simulink model "sampleModel1479_sub_sub"  (R2023a)
settings: Solver=VariableStepAuto  StartTime=0.0  StopTime=10.0  RelTol=1e-3
libraries: hdlsllib x6
settings Model: Creator=user1  LastModifiedBy=user1
settings OptimizationCC: BlockReduction=off  ConditionallyExecuteInputs=off

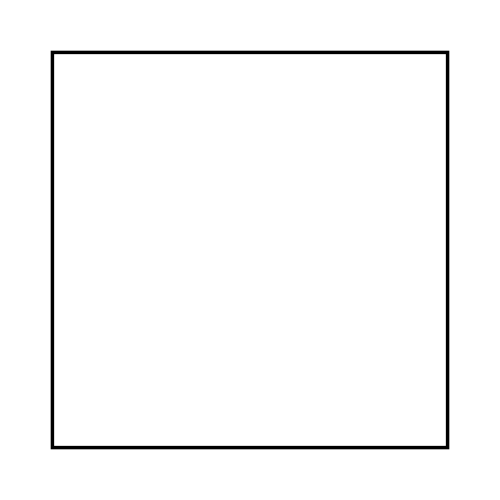
[thumbnail: Simulink's stored preview of the top-level diagram]
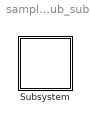
== system sampleModel1479_sub_sub ==
  Subsystem : Subsystem

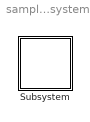
== system sampleModel1479_sub_sub/Subsystem ==
  Subsystem : Subsystem

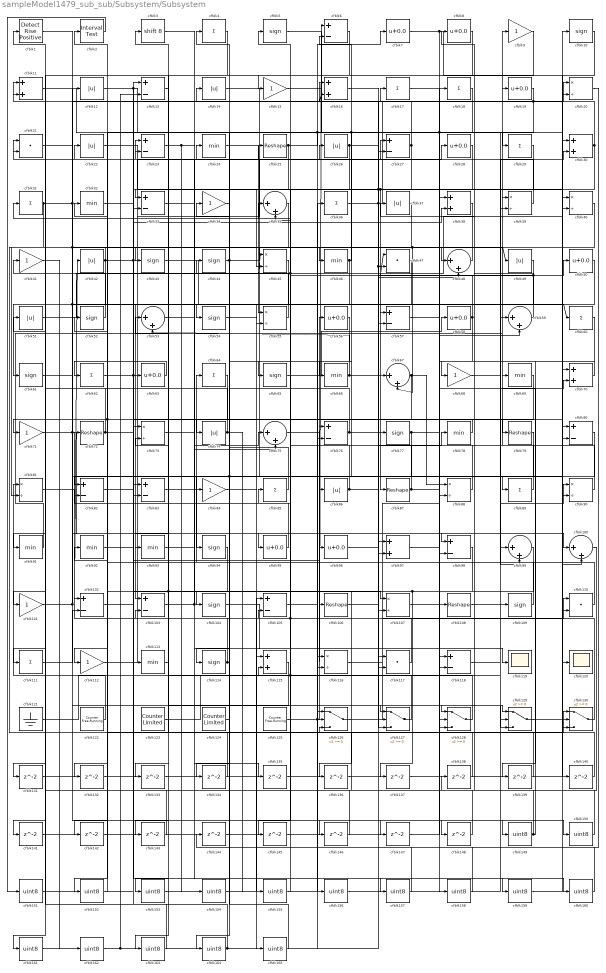
== system sampleModel1479_sub_sub/Subsystem/Subsystem ==
  cfblk1 : hdlsllib/Logic and Bit Operations/Detect Rise Positive  vinit=0  OutDataTypeStr=uint8
  cfblk{5,10,43..44,52,54,61,65,77,94,104,109,114} (13 alike) : Signum
  cfblk{35,48,53,59,67,75,99..100} (8 alike) : Sum  Inputs=|++  OutDataTypeStr=uint8
  cfblk{9,15,34,41,68,71,84,101,112} (9 alike) : Gain  OutDataTypeStr=uint8
  cfblk{6,13,23,27,33,57,76,80,82..83,98,102..103,105,118} (15 alike) : Sum  Inputs=+-  OutDataTypeStr=uint8
  cfblk{25,72,79,87,106,108} (6 alike) : Reshape
  cfblk{20,39..40,45,55,73,81,88,90,107,116} (11 alike) : Product  Inputs=*/  OutDataTypeStr=uint8  RndMeth=Zero  SaturateOnIntegerOverflow=on
  cfblk{11,16,30,38,70,97,115} (7 alike) : Sum  OutDataTypeStr=uint8
  cfblk{21,47,110,117} (4 alike) : DotProduct  OutDataTypeStr=uint8
  cfblk{4,17..18,29,31,36,60,62,64,85,89,111} (12 alike) : Sum  Inputs=+  OutDataTypeStr=uint8
  cfblk{24,32,46,66,69,78,91..93,113} (10 alike) : MinMax  OutDataTypeStr=uint8
  cfblk119 : Scope
  cfblk{12,14,22,26,37,42,49,51,74,86} (10 alike) : Abs  OutDataTypeStr=uint8  SaturateOnIntegerOverflow=off
  cfblk120 : Scope
  cfblk121 : Ground
  cfblk122 : hdlsllib/Sources/Counter Free-Running  NumBits=16  tsamp=-1
  cfblk123 : hdlsllib/Sources/Counter Limited  uplimit=7  tsamp=-1
  cfblk124 : hdlsllib/Sources/Counter Limited  uplimit=7  tsamp=-1
  cfblk125 : hdlsllib/Sources/Counter Free-Running  NumBits=16  tsamp=-1
  cfblk{126..130} (5 alike) : Switch  OutDataTypeStr=uint8  SaturateOnIntegerOverflow=off  InputSameDT=off
  cfblk{131..148} (18 alike) : Delay  SampleTime=1
  cfblk{149..165} (17 alike) : DataTypeConversion  OutDataTypeStr=uint8  SaturateOnIntegerOverflow=off  RndMeth=Floor
  cfblk{7..8,19,28,50,56,58,63,95..96} (10 alike) : Bias  Bias=0.0  SaturateOnIntegerOverflow=off
  cfblk2 : hdlsllib/Logic and Bit Operations/Interval Test  IntervalClosedRight=on  uplimit=0.5  IntervalClosedLeft=on  lowlimit=-0.5  OutDataTypeStr=uint8
  cfblk3 : ArithShift  BitShiftNumber=8
  wires:
  cfblk165/1 -> cfblk34/1
  cfblk54/1 -> cfblk165/1
  cfblk164/1 -> cfblk27/2, cfblk13/1
  cfblk163/1 -> cfblk41/1
  cfblk162/1 -> cfblk116/2, cfblk13/2
  cfblk161/1 -> cfblk97/2
  cfblk160/1 -> cfblk97/1
  cfblk73/1 -> cfblk160/1
  cfblk159/1 -> cfblk40/2
  cfblk97/1 -> cfblk159/1
  cfblk158/1 -> cfblk105/2
  cfblk104/1 -> cfblk158/1
  cfblk157/1 -> cfblk105/1
  cfblk32/1 -> cfblk157/1
  cfblk156/1 -> cfblk109/1
  cfblk105/1 -> cfblk156/1
  cfblk155/1 -> cfblk115/2
  cfblk154/1 -> cfblk115/1
  cfblk153/1 -> cfblk116/1
  cfblk115/1 -> cfblk153/1
  cfblk152/1 -> cfblk2/1
  cfblk37/1 -> cfblk152/1
  cfblk151/1 -> cfblk63/1
  cfblk2/1 -> cfblk151/1
  cfblk150/1 -> cfblk1/1
  cfblk147/1 -> cfblk150/1
  cfblk149/1 -> cfblk8/1, cfblk69/1
  cfblk148/1 -> cfblk126/3
  cfblk84/1 -> cfblk147/1
  cfblk146/1 -> cfblk73/1
  cfblk92/1 -> cfblk146/1
  cfblk145/1 -> cfblk88/2
  cfblk144/1 -> cfblk38/1
  cfblk20/1 -> cfblk144/1
  cfblk143/1 -> cfblk83/1
  cfblk13/1 -> cfblk143/1
  cfblk142/1 -> cfblk98/2
  cfblk141/1 -> cfblk67/1
  cfblk6/1 -> cfblk141/1
  cfblk140/1 -> cfblk126/1
  cfblk129/1 -> cfblk140/1
  cfblk139/1 -> cfblk103/2
  cfblk60/1 -> cfblk139/1
  cfblk138/1 -> cfblk35/2
  cfblk100/1 -> cfblk138/1
  cfblk137/1 -> cfblk110/2
  cfblk136/1 -> cfblk30/1
  cfblk135/1 -> cfblk70/1
  cfblk53/1 -> cfblk135/1
  cfblk134/1 -> cfblk82/2
  cfblk133/1 -> cfblk39/2
  cfblk132/1 -> cfblk40/1
  cfblk18/1 -> cfblk132/1
  cfblk131/1 -> cfblk57/2
  cfblk52/1 -> cfblk21/2
  cfblk118/1 -> cfblk99/1
  cfblk103/1 -> cfblk27/1, cfblk127/3
  cfblk19/1 -> cfblk76/2, cfblk54/1, cfblk86/1, cfblk16/2
  cfblk80/1 -> cfblk133/1, cfblk134/1
  cfblk124/1 -> cfblk44/1
  cfblk67/1 -> cfblk88/1, cfblk131/1
  cfblk4/1 -> cfblk43/1
  cfblk15/1 -> cfblk118/1, cfblk99/2
  cfblk58/1 -> cfblk25/1, cfblk128/2
  cfblk31/1 -> cfblk84/1, cfblk49/1, cfblk16/1, cfblk81/2
  cfblk111/1 -> cfblk102/2
  cfblk75/1 -> cfblk76/1
  cfblk10/1 -> cfblk130/3
  cfblk69/1 -> cfblk112/1, cfblk161/1
  cfblk46/1 -> cfblk6/2, cfblk83/2
  cfblk28/1 -> cfblk47/2, cfblk117/2, cfblk126/2
  cfblk79/1 -> cfblk82/1
  cfblk114/1 -> cfblk14/1, cfblk92/1
  cfblk41/1 -> cfblk162/1
  cfblk35/1 -> cfblk111/1
  cfblk126/1 -> cfblk110/1
  cfblk68/1 -> cfblk30/2
  cfblk107/1 -> cfblk129/1
  cfblk36/1 -> cfblk19/1, cfblk118/2
  cfblk48/1 -> cfblk46/1
  cfblk106/1 -> cfblk20/1
  cfblk3/1 -> cfblk107/1
  cfblk78/1 -> cfblk71/1
  cfblk7/1 -> cfblk100/2, cfblk129/3
  cfblk23/1 -> cfblk75/2, cfblk154/1
  cfblk5/1 -> cfblk120/1
  cfblk61/1 -> cfblk100/1
  cfblk17/1 -> cfblk108/1
  cfblk70/1 -> cfblk68/1
  cfblk43/1 -> cfblk55/2
  cfblk98/1 -> cfblk114/1
  cfblk40/1 -> cfblk67/2, cfblk66/1
  cfblk21/1 -> cfblk60/1, cfblk128/3
  cfblk101/1 -> cfblk12/1, cfblk148/1
  cfblk57/1 -> cfblk79/1
  cfblk108/1 -> cfblk90/1
  cfblk22/1 -> cfblk80/1, cfblk117/1
  cfblk66/1 -> cfblk53/2, cfblk128/1
  cfblk94/1 -> cfblk142/1, cfblk163/1
  cfblk109/1 -> cfblk52/1
  cfblk25/1 -> cfblk7/1, cfblk45/2
  cfblk45/1 -> cfblk74/1
  cfblk113/1 -> cfblk73/2
  cfblk16/1 -> cfblk98/1
  cfblk130/1 -> cfblk53/1
  cfblk81/1 -> cfblk102/1
  cfblk99/1 -> cfblk136/1, cfblk137/1
  cfblk59/1 -> cfblk47/1, cfblk37/1
  cfblk82/1 -> cfblk113/1
  cfblk27/1 -> cfblk11/2, cfblk127/2
  cfblk34/1 -> cfblk164/1
  cfblk85/1 -> cfblk4/1
  cfblk49/1 -> cfblk65/1
  cfblk11/1 -> cfblk130/2
  cfblk9/1 -> cfblk15/1
  cfblk96/1 -> cfblk50/1
  cfblk1/1 -> cfblk149/1
  cfblk93/1 -> cfblk75/1
  cfblk88/1 -> cfblk31/1
  cfblk74/1 -> cfblk51/1, cfblk155/1
  cfblk77/1 -> cfblk70/2, cfblk107/2
  cfblk86/1 -> cfblk78/1, cfblk23/2
  cfblk102/1 -> cfblk96/1
  cfblk72/1 -> cfblk11/1, cfblk90/2
  cfblk63/1 -> cfblk62/1
  cfblk76/1 -> cfblk77/1, cfblk24/1
  cfblk29/1 -> cfblk57/1, cfblk33/2
  cfblk87/1 -> cfblk35/1, cfblk59/2
  cfblk62/1 -> cfblk26/1, cfblk20/2
  cfblk24/1 -> cfblk55/1
  cfblk30/1 -> cfblk17/1, cfblk145/1
  cfblk26/1 -> cfblk33/1, cfblk48/2
  cfblk123/1 -> cfblk59/1
  cfblk95/1 -> cfblk72/1
  cfblk51/1 -> cfblk10/1
  cfblk65/1 -> cfblk58/1
  cfblk64/1 -> cfblk101/1
  cfblk33/1 -> cfblk119/1
  cfblk55/1 -> cfblk32/1
  cfblk89/1 -> cfblk23/1
  cfblk116/1 -> cfblk18/1
  cfblk8/1 -> cfblk93/1
  cfblk50/1 -> cfblk61/1
  cfblk12/1 -> cfblk29/1, cfblk80/2
  cfblk121/1 -> cfblk36/1
  cfblk83/1 -> cfblk94/1
  cfblk39/1 -> cfblk22/1
  cfblk128/1 -> cfblk5/1, cfblk45/1, cfblk3/1
  cfblk127/1 -> cfblk56/1
  cfblk47/1 -> cfblk103/1
  cfblk38/1 -> cfblk87/1
  cfblk90/1 -> cfblk39/1
  cfblk14/1 -> cfblk89/1
  cfblk112/1 -> cfblk28/1
  cfblk42/1 -> cfblk38/2, cfblk106/1, cfblk130/1, cfblk91/1
  cfblk125/1 -> cfblk6/1, cfblk127/1
  cfblk56/1 -> cfblk104/1
  cfblk117/1 -> cfblk42/1, cfblk85/1
  cfblk122/1 -> cfblk81/1
  cfblk91/1 -> cfblk9/1
  cfblk71/1 -> cfblk95/1, cfblk129/2
  cfblk44/1 -> cfblk21/1, cfblk48/1
  cfblk110/1 -> cfblk64/1
